simulink library "headingSetpointCalculation_cl"  (R2018b)
settings: Solver=VariableStepAuto  StartTime=0.0  StopTime=10.0  RelTol=1e-3
undefined symbols (not defined in the file or in its folder): initialPathPosition_none
libraries: flatlandHeading_ul x1, offsetLeadDistance_ul x1, pathPosition_ul x1, pathProjection_ul x1
settings Model: Creator=mcobb  LastModifiedBy=mcobb
settings DebuggingCC: LibraryContextMissingDiagnostic=none
settings SFSimCC: SimUseLocalCustomCode=off
settings RTWCC: RTWUseLocalCustomCode=off

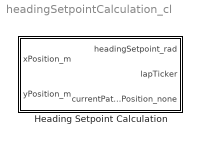
== system headingSetpointCalculation_cl ==
  Heading Setpoint Calculation : Subsystem

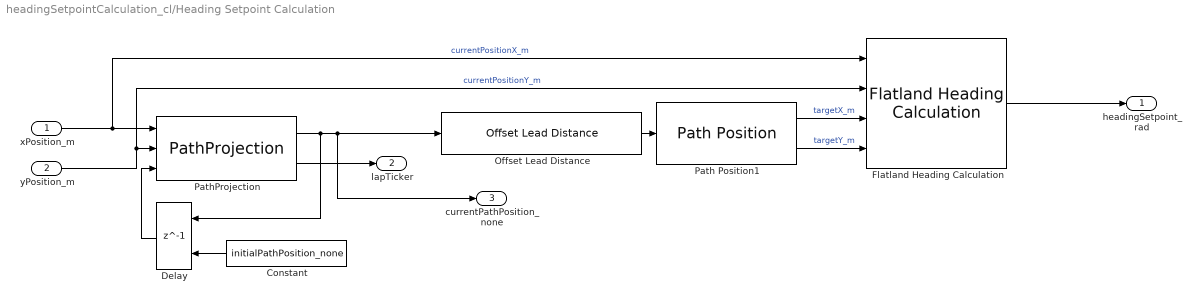
== system headingSetpointCalculation_cl/Heading Setpoint Calculation ==
  xPosition_m : Inport
  yPosition_m : Inport  Port=2
  Constant : Constant  Value=initialPathPosition_none
  Delay : Delay  DelayLength=1  InitialConditionSource=Input port  InitialCondition=0
      settings: InputPortMap=u0,p4
  Flatland Heading Calculation : flatlandHeading_ul/Flatland Heading Calculation  SystemSampleTime=-1
  Offset Lead Distance : offsetLeadDistance_ul/Offset Lead Distance  SystemSampleTime=-1
  Path Position1 : pathPosition_ul/Path Position  SystemSampleTime=-1
  PathProjection : pathProjection_ul/PathProjection  SystemSampleTime=-1
  headingSetpoint_rad : Outport
  lapTicker : Outport  Port=2
  currentPathPosition_none : Outport  Port=3
  wires:
  Offset Lead Distance/1 -> Path Position1/1
  Flatland Heading Calculation/1 -> headingSetpoint_rad/1
  PathProjection/1 -> Delay/1, currentPathPosition_none/1, Offset Lead Distance/1
  Path Position1/1 -> Flatland Heading Calculation/3  "targetX_m"
  Path Position1/2 -> Flatland Heading Calculation/4  "targetY_m"
  xPosition_m/1 -> PathProjection/1, Flatland Heading Calculation/1  "currentPositionX_m"
  yPosition_m/1 -> Flatland Heading Calculation/2, PathProjection/2  "currentPositionY_m"
  Delay/1 -> PathProjection/3
  Constant/1 -> Delay/2
  PathProjection/2 -> lapTicker/1
